simulink model "CO2_Insufflator"  (R2024b)
settings: Solver=VariableStepAuto  StartTime=0.0  StopTime=250  RelTol=1e-3
libraries: fl_lib x23, nesl_utility x9, SimscapeFluids_lib x6, slpidlib x2
(part 1 of 3)
settings Model: Creator=nafis  LastModifiedBy=nafis
settings SolverCC: DateTimeAtSimulationTimeZero=[]
settings DebuggingCC: AlgebraicLoopMsg=none

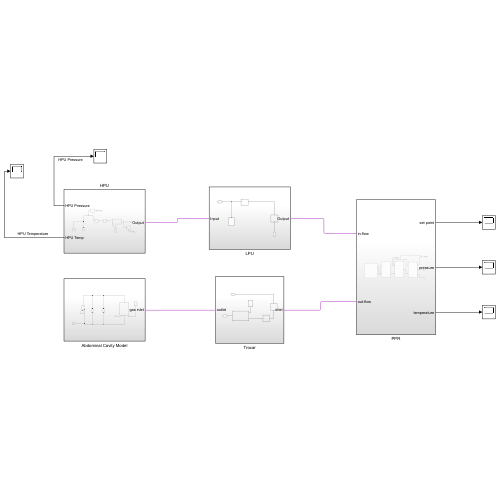
[thumbnail: Simulink's stored preview of the top-level diagram]
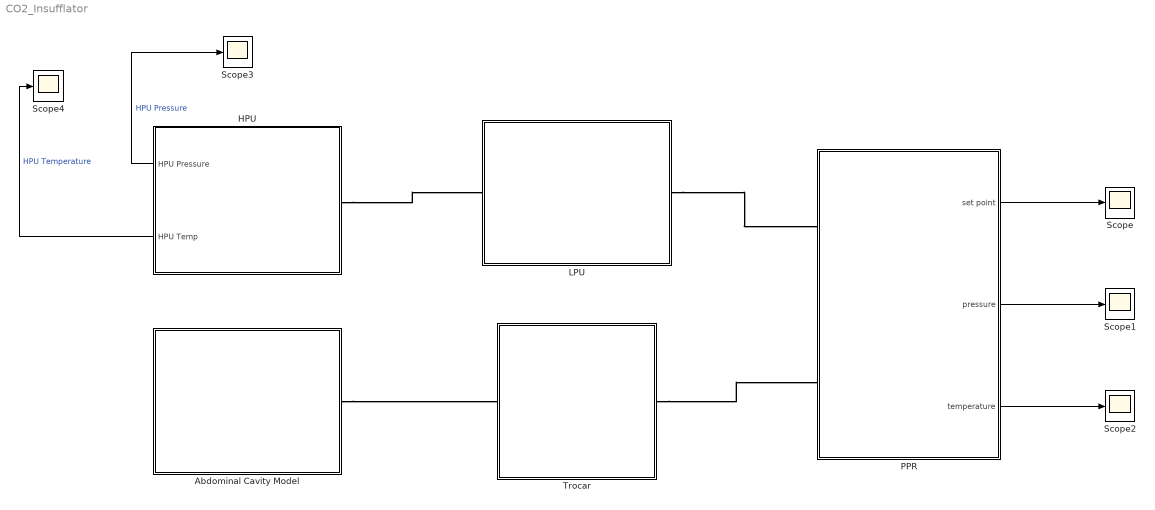
== system CO2_Insufflator ==
  Abdominal Cavity Model : Subsystem
  HPU : Subsystem
  LPU : Subsystem
  PPR : Subsystem
  Scope{,1..4} (5 alike) : Scope
  Trocar : Subsystem
  wires:
  PPR/3(temperature) -> Scope2/1
  PPR/2(pressure) -> Scope1/1
  PPR/1(set point) -> Scope/1
  HPU/1(HPU Pressure) -> Scope3/1  "HPU Pressure"
  HPU/2(HPU Temp) -> Scope4/1  "HPU Temperature"
  connections:
  HPU/LConn1 -- LPU/LConn1
  LPU/RConn1 -- PPR/LConn1
  Trocar/RConn1 -- PPR/LConn2
  Abdominal Cavity Model/RConn1 -- Trocar/LConn1

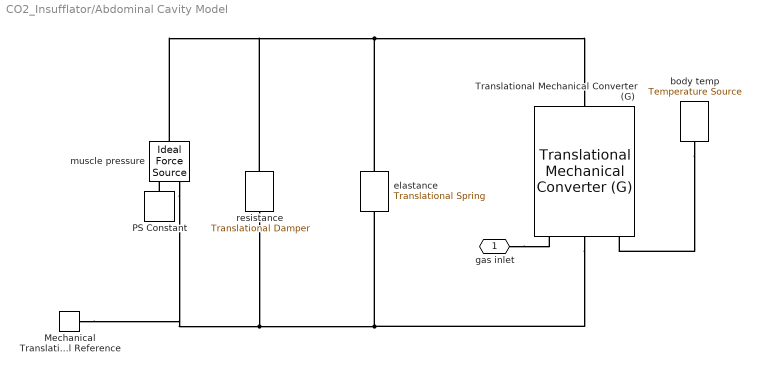
== system CO2_Insufflator/Abdominal Cavity Model ==
  Mechanical Translational Reference : fl_lib/Mechanical/Translational Elements/Mechanical Translational Reference
  PS Constant : fl_lib/Physical Signals/Sources/PS Constant  constant=1
  Translational Mechanical Converter (G) : fl_lib/Gas/Elements/Translational Mechanical Converter (G)  mech_orientation=foundation.enum.MechOrientationTranslational.Positive  displacement_spec=foundation.enum.DisplacementSpec.Calculate  length_init=0 m  interface_area=1 m^2  dead_volume=1e-5 m^3  area_A=0.01 m^2  environment_spec=foundation.enum.pressure_spec.atmospheric  environment_pressure=0.101325 MPa  p_I_specify=off  p_I_priority=High  p_I=0.101325 MPa  p_I_nominal_specify=off  p_I_nominal_value=1  p_I_nominal_unit=MPa  T_I_specify=off  T_I_priority=High  T_I=293.15 K  T_I_nominal_specify=off  T_I_nominal_value=1  T_I_nominal_unit=K  rho_I_specify=off  rho_I_priority=None  rho_I=1.2 kg/m^3  rho_I_nominal_specify=off  rho_I_nominal_value=1  rho_I_nominal_unit=kg/m^3
      settings: InternalSimscapePortConfiguration="{\"Bottom\":[],\"Left\":[{\"id\":\"A\",\"label\":\"A\",\"type\":\"foundation.gas.gas\"},{\"id\":\"C\",\"label\":\"C\",\"type\":\"foundation.mechanical.translational.translational\"},{\"id\":\"H\",\"label\":\"H\",\"type\":\"foundation.thermal.thermal\"}],\"Right\":[{\"id\":\"R\",\"label\":\"R\",\"type\":\"foundation.mechanical.translational.translational\"}],\"Top\":[]}"
  body temp : fl_lib/Thermal/Thermal Sources/Temperature Source  temperature=37 degC
  elastance : fl_lib/Mechanical/Translational Elements/Translational Spring  spr_rate=1250 N/m  v_specify=off  v_priority=None  v=0 m/s  v_nominal_specify=off  v_nominal_value=1  v_nominal_unit=m/s  f_specify=off  f_priority=None  f=0 N  f_nominal_specify=off  f_nominal_value=1  f_nominal_unit=N  x_specify=off  x_priority=High  x=0 m  x_nominal_specify=off  x_nominal_value=1  x_nominal_unit=m
  muscle pressure : fl_lib/Mechanical/Mechanical Sources/Ideal Force Source
  resistance : fl_lib/Mechanical/Translational Elements/Translational Damper  D=0.1 N*s/m  v_specify=off  v_priority=None  v=0 m/s  v_nominal_specify=off  v_nominal_value=1  v_nominal_unit=m/s  f_specify=off  f_priority=None  f=0 N  f_nominal_specify=off  f_nominal_value=1  f_nominal_unit=N
  gas inlet : PMIOPort  Side=Right
  connections:
  gas inlet/RConn1 -- Translational Mechanical Converter (G)/LConn1
  body temp/LConn1 -- Translational Mechanical Converter (G)/LConn3
  elastance/LConn1 -- muscle pressure/LConn1 -- resistance/LConn1 -- Translational Mechanical Converter (G)/RConn1
  Translational Mechanical Converter (G)/LConn2 -- muscle pressure/RConn2 -- Mechanical Translational Reference/LConn1 -- resistance/RConn1 -- elastance/RConn1
  PS Constant/RConn1 -- muscle pressure/RConn1
